simulink model "exp10_2_3"  (R2020a)
settings: Solver=VariableStepAuto  StartTime=0.0  StopTime=160  RelTol=1e-3
libraries: simulink x1
settings Model: Creator=zengw  LastModifiedBy=zengw

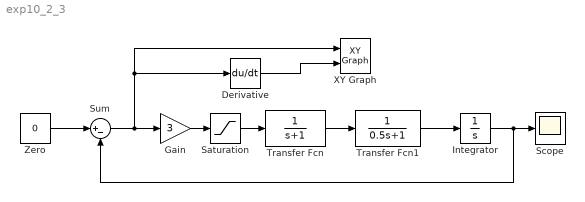
== system exp10_2_3 ==
  Derivative : Derivative
  Gain : Gain  Gain=3
  Integrator : Integrator  InitialCondition=1.5
  Saturation : Saturate  UpperLimit=3.6  LowerLimit=-3.6
  Scope : Scope
  Sum : Sum  Inputs=|+-
  Transfer Fcn : TransferFcn  Denominator=[1 1]
  Transfer Fcn1 : TransferFcn  Denominator=[0.5 1]
  XY Graph : simulink/Sinks/XY Graph  xmin=-3  xmax=3  ymin=-3  ymax=3  st=0.1
  Zero : Constant  Value=0  OutDataTypeStr=Inherit: Inherit via back propagation
  wires:
  Zero/1 -> Sum/1
  Sum/1 -> Gain/1, Derivative/1, XY Graph/1
  Saturation/1 -> Transfer Fcn/1
  Transfer Fcn/1 -> Transfer Fcn1/1
  Transfer Fcn1/1 -> Integrator/1
  Integrator/1 -> Sum/2, Scope/1
  Derivative/1 -> XY Graph/2
  Gain/1 -> Saturation/1
